simulink model "uz_pmsm_model_nonlinear"  (R2023a)
settings: Solver=FixedStepAuto  StartTime=0.0  StopTime=0.5  RelTol=1e-3
PreLoadFcn:
  | uz_pmsm_model_init_parameter
PostLoadFcn:
  | % Import the data from Excel for a lookup table
  | FluxMapData = readtable('C:\Users\Philipp\ultrazohm\ultrazohm_sw\ip_cores\uz_pmsm_model\FluxMapData_2023-05-26_13-07-57.csv');
  | % Row indices for lookup table
  | d_current_in_d_axis = FluxMapData(8:27,1:end);
  | % Column indices for lookup table
  | q_current_in_d_axis = FluxMapData(29:48,1:end);
  | % Output values for lookup table
  | d_Flux_d_axis = FluxMapData(50:69,1:end);
values from neighbouring files (symbols this model uses):
  d_current_d_Flux = FluxMapData{1,:}    [uz_pmsm_model_nonlinear_init_parameter.m]
  d_current_q_Flux = FluxMapData{66,:}    [uz_pmsm_model_nonlinear_init_parameter.m]
  Flux_d = FluxMapData{43:62,:}'*(1e-3)    [uz_pmsm_model_nonlinear_init_parameter.m]
  Flux_q = FluxMapData{108:end,:}'*(1e-3)    [uz_pmsm_model_nonlinear_init_parameter.m]
  friction_coefficient = 0.001    [uz_pmsm_model_nonlinear_init_parameter.m]
  inertia = 0.001    [uz_pmsm_model_nonlinear_init_parameter.m]
  k_i_d = R_1/(2*tau_sum)    (= 2812.5)    [uz_pmsm_model_nonlinear_init_parameter.m]
  k_p_d = L_d/(2*tau_sum)    (= 10.9375)    [uz_pmsm_model_nonlinear_init_parameter.m]
  k_p_q = L_q/(2*tau_sum)    (= 10.9375)    [uz_pmsm_model_nonlinear_init_parameter.m]
  L_d = 1.75e-3    (= 0.00175)    [uz_pmsm_model_nonlinear_init_parameter.m]
  L_q = 1.75e-3    (= 0.00175)    [uz_pmsm_model_nonlinear_init_parameter.m]
  polepair = 4    [uz_pmsm_model_nonlinear_init_parameter.m]
  psi_pm = 0.042    [uz_pmsm_model_nonlinear_init_parameter.m]
  q_current_d_Flux = FluxMapData{22:41,1}    [uz_pmsm_model_nonlinear_init_parameter.m]
  q_current_q_Flux = FluxMapData{87:106,1}    [uz_pmsm_model_nonlinear_init_parameter.m]
  R_1 = 0.45    [uz_pmsm_model_nonlinear_init_parameter.m]
  setpoint_step = 10.0    (= 10)    [compare_simulation_to_measurement.m]    (also in uz_pmsm_model_nonlinear_init_parameter.m)
  simulate_mechanical = true    [compare_simulation_to_measurement.m]    (also in uz_pmsm_model_nonlinear_init_parameter.m = false)
  simulate_open_loop = true    [compare_simulation_to_measurement.m]    (also in uz_pmsm_model_nonlinear_init_parameter.m)
  static_friction_torque = 0.01    [uz_pmsm_model_nonlinear_init_parameter.m]
  ts = 1/5e5    (= 2e-06)    [uz_pmsm_model_nonlinear_init_parameter.m]
undefined symbols (not defined in the file or in its folder): Ldd, Ldq, Lqd, Lqq
libraries: slpidlib x2
settings Model: DataTypeOverride=Off  Creator=ts  LastModifiedBy=Philipp
settings SolverCC: AlgebraicLoopSolver=TrustRegion  AutoInsertRateTranBlk=on
settings DataIOCC: LimitDataPoints=on  SaveOutput=off  SaveTime=off
settings OptimizationCC: BlockReduction=off  ConditionallyExecuteInputs=off  DefaultParameterBehavior=Inlined  LifeSpan=inf
settings DebuggingCC: AlgebraicLoopMsg=error  SingleTaskRateTransMsg=error  UnconnectedInputMsg=warning  UnconnectedOutputMsg=warning  UnconnectedLineMsg=warning  AllowSymbolicDim=off  StrictBusMsg=ErrorOnBusTreatedAsVector  SFUnexpectedBacktrackingDiag=warning  SFNoUnconditionalDefaultTransitionDiag=warning  SFExecutionAtInitializationDiag=none  ArithmeticOperatorsInVariantConditions=warning
settings HardwareCC: ProdBitPerPointer=32  ProdBitPerSizeT=32  ProdBitPerPtrDiffT=32  ProdLargestAtomicFloat=None  ProdIntDivRoundTo=Undefined  ProdEndianess=Unspecified  ProdWordSize=32  ProdHWDeviceType=ASIC/FPGA->ASIC/FPGA  ProdEqTarget=off
settings ModelReferenceCC: EnableRefExpFcnMdlSchedulingChecks=on
settings SFSimCC: SimUseLocalCustomCode=off  CustomCodeUndefinedFunction=UseInterfaceOnly
settings RTWCC: RTWUseLocalCustomCode=off  DLArmComputeVersion=19.05
settings CodeAppCC: StateflowObjectComments=on
settings GRTTargetCC: TargetLangStandard=C89/C90 (ANSI)
settings ConfigComp: CovScope=ReferencedModels  CovMetricSettings=dw  CovSaveCumulativeToWorkspaceVar=on  CovSaveSingleToWorkspaceVar=on  CovExternalEMLEnable=off  CovSFcnEnable=off

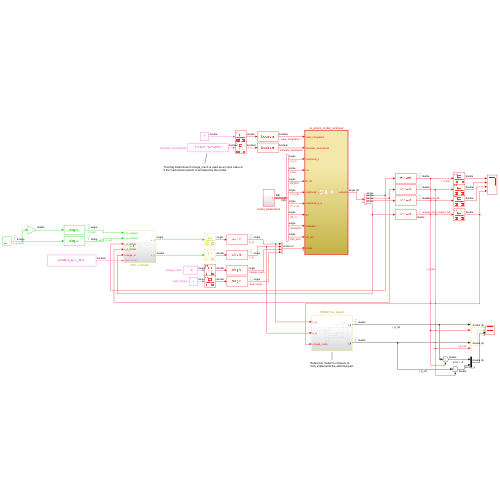
[thumbnail: Simulink's stored preview of the top-level diagram]
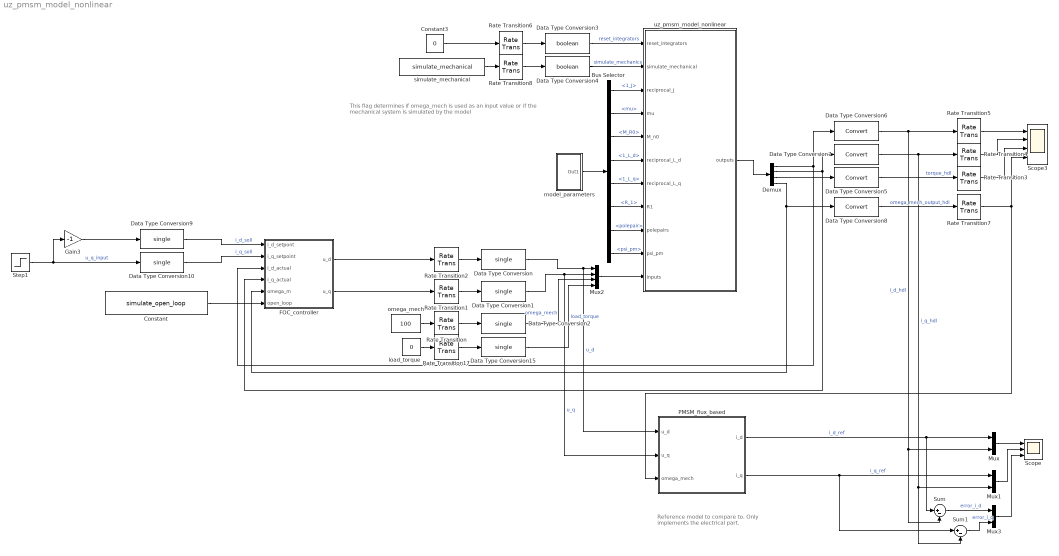
== system uz_pmsm_model_nonlinear ==
  note: Reference model to compare to.
      | Only implements the electrical part.
  note: This flag determines if omega_mech is used as an input value or
      | if the mechanical system is simulated by the model
  Bus Selector : BusSelector  OutputSignals=1_J,mu,M_R0,1_L_d,1_L_q,R_1,polepair,psi_pm
  Constant : Constant  Value=simulate_open_loop
  Constant3 : Constant  Value=0
  Data Type Conversion{,1..2,9..10,15} (6 alike) : DataTypeConversion  OutDataTypeStr=single  SaturateOnIntegerOverflow=off  RndMeth=Floor
  Data Type Conversion3 : DataTypeConversion  OutDataTypeStr=boolean  SaturateOnIntegerOverflow=off  RndMeth=Floor
  Data Type Conversion4 : DataTypeConversion  OutDataTypeStr=boolean  SaturateOnIntegerOverflow=off  RndMeth=Floor
  Data Type Conversion{5..8} (4 alike) : DataTypeConversion  SaturateOnIntegerOverflow=off  RndMeth=Floor
  Demux : Demux
  FOC_controller : Subsystem
  Gain3 : Gain  Gain=-1
  Mux : Mux  Inputs=2
  Mux1 : Mux  Inputs=2
  Mux2 : Mux
  Mux3 : Mux  Inputs=2
  PMSM_flux_based : Subsystem
  Rate Transition{,1..2,6,8,17} (6 alike) : RateTransition  OutPortSampleTime=ts
  Rate Transition{3..5,7} (4 alike) : RateTransition
  Scope : Scope  NumInputPorts=3
  Scope3 : Scope  NumInputPorts=4
  Step1 : Step  Time=0.2  After=setpoint_step
  Sum : Sum  Inputs=|+-
  Sum1 : Sum  Inputs=|+-
  load_torque : Constant  Value=0
  model_parameters : Subsystem
  omega_mech : Constant  Value=100
  simulate_mechanical : Constant  Value=simulate_mechanical
  uz_pmsm_model_nonlinear : Subsystem  TreatAsAtomicUnit=on
  wires:
  Rate Transition/1 -> Data Type Conversion2/1
  Rate Transition1/1 -> Data Type Conversion1/1
  Rate Transition2/1 -> Data Type Conversion/1
  Data Type Conversion6/1 -> Mux/2, Sum/2, Rate Transition5/1  "i_d_hdl"
  Data Type Conversion7/1 -> Rate Transition4/1, Mux1/2, Sum1/2  "i_q_hdl"
  Data Type Conversion5/1 -> Rate Transition3/1  "torque_hdl"
  Rate Transition4/1 -> Scope3/2
  Rate Transition5/1 -> Scope3/1
  Rate Transition3/1 -> Scope3/3
  Rate Transition6/1 -> Data Type Conversion3/1
  Constant3/1 -> Rate Transition6/1
  Rate Transition8/1 -> Data Type Conversion4/1
  simulate_mechanical/1 -> Rate Transition8/1
  Data Type Conversion3/1 -> uz_pmsm_model_nonlinear/1(reset_integrators)  "reset_integrators"
  Data Type Conversion4/1 -> uz_pmsm_model_nonlinear/2(simulate_mechanical)  "simulate_mechanics"
  load_torque/1 -> Rate Transition17/1
  Rate Transition17/1 -> Data Type Conversion15/1
  Mux/1 -> Scope/1
  Mux1/1 -> Scope/2
  PMSM_flux_based/2(i_q) -> Mux1/1, Sum1/1  "i_q_ref"
  PMSM_flux_based/1(i_d) -> Mux/1, Sum/1  "i_d_ref"
  Data Type Conversion8/1 -> Rate Transition7/1  "omega_mech_output_hdl"
  Rate Transition7/1 -> PMSM_flux_based/3(omega_mech), Scope3/4
  Bus Selector/1 -> uz_pmsm_model_nonlinear/3(reciprocal_J)  "<1_J>"
  Bus Selector/2 -> uz_pmsm_model_nonlinear/4(mu)  "<mu>"
  Bus Selector/3 -> uz_pmsm_model_nonlinear/5(M_n0)  "<M_R0>"
  Bus Selector/4 -> uz_pmsm_model_nonlinear/6(reciprocal_L_d)  "<1_L_d>"
  Bus Selector/5 -> uz_pmsm_model_nonlinear/7(reciprocal_L_q)  "<1_L_q>"
  Bus Selector/6 -> uz_pmsm_model_nonlinear/8(R1)  "<R_1>"
  Bus Selector/7 -> uz_pmsm_model_nonlinear/9(polepairs)  "<polepair>"
  Bus Selector/8 -> uz_pmsm_model_nonlinear/10(psi_pm)  "<psi_pm>"
  model_parameters/1(Out1) -> Bus Selector/1
  Sum/1 -> Mux3/1  "error_i_d"
  Sum1/1 -> Mux3/2  "error_i_q"
  Mux3/1 -> Scope/3
  Step1/1 -> Gain3/1, Data Type Conversion10/1  "u_q_input"
  Demux/3 -> Data Type Conversion5/1
  Gain3/1 -> Data Type Conversion9/1
  Demux/1 -> Data Type Conversion6/1, FOC_controller/3(i_d_actual)
  Demux/4 -> Data Type Conversion8/1, FOC_controller/5(omega_m)
  Demux/2 -> Data Type Conversion7/1, FOC_controller/4(i_q_actual)
  Data Type Conversion/1 -> PMSM_flux_based/1(u_d), Mux2/1  "u_d"
  Data Type Conversion1/1 -> PMSM_flux_based/2(u_q), Mux2/2  "u_q"
  Data Type Conversion15/1 -> Mux2/4  "load_torque"
  Data Type Conversion2/1 -> Mux2/3  "omega_mech"
  Mux2/1 -> uz_pmsm_model_nonlinear/11(inputs)
  uz_pmsm_model_nonlinear/1(outputs) -> Demux/1
  Data Type Conversion9/1 -> FOC_controller/1(i_d_setpont)  "i_d_soll"
  Data Type Conversion10/1 -> FOC_controller/2(i_q_setpoint)  "i_q_soll"
  FOC_controller/1(u_d) -> Rate Transition2/1
  FOC_controller/2(u_q) -> Rate Transition1/1
  omega_mech/1 -> Rate Transition/1
  Constant/1 -> FOC_controller/6(open_loop)

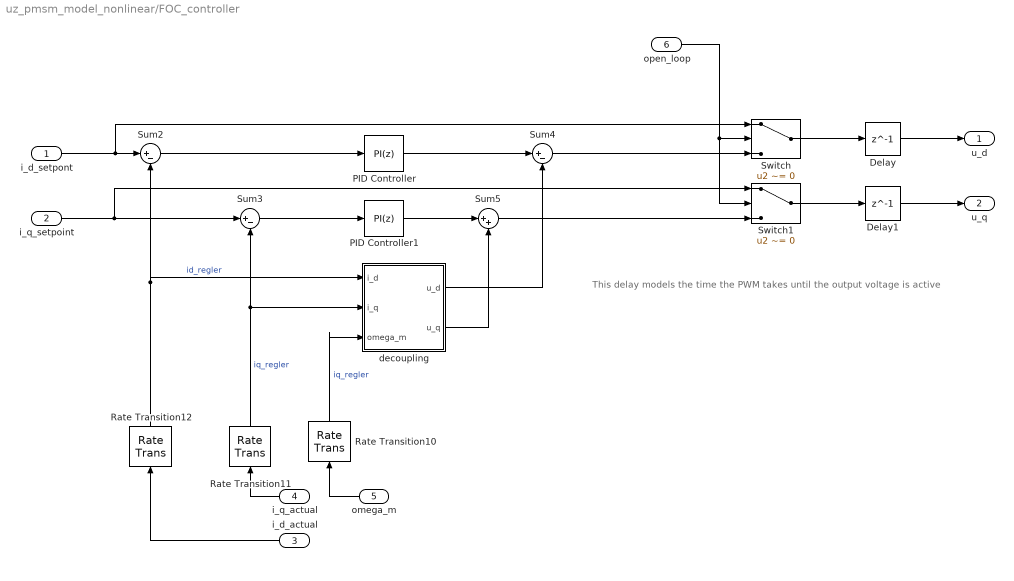
== system uz_pmsm_model_nonlinear/FOC_controller ==
  note: This delay models the time the PWM takes until the output voltage is active
  i_d_setpont : Inport
  i_q_setpoint : Inport  Port=2
  i_d_actual : Inport  Port=3
  i_q_actual : Inport  Port=4
  omega_m : Inport  Port=5
  open_loop : Inport  Port=6
  Delay : Delay  DelayLength=1
  Delay1 : Delay  DelayLength=1
  PID Controller : slpidlib/PID Controller  Controller=PI  Form=Parallel  TimeDomain=Discrete-time  UseExternalTs=off  SampleTime=-1  IntegratorMethod=Forward Euler  FilterMethod=Forward Euler  ControllerParametersSource=internal  P=k_p_d  I=k_i_d  UseKiTs=off  D=0  N=100  UseFilter=on  TunerSelectOption=Transfer Function Based (PID Tuner App)  InitialConditionSource=internal  InitialConditionForIntegrator=0  InitialConditionForFilter=0  DifferentiatorICPrevScaledInput=0  ExternalReset=none  TrackingMode=off  Kt=1  LimitOutput=off  SatLimitsSource=internal  UpperSaturationLimit=inf  LowerSaturationLimit=-inf  LinearizeAsGain=on  AntiWindupMode=none  Kb=1  LimitIntegrator=off  UpperIntegratorSaturationLimit=inf  LowerIntegratorSaturationLimit=-inf  POutMin=[]  POutMax=[]  IOutMin=[]  IOutMax=[]  DOutMin=[]  DOutMax=[]  NOutMin=[]  NOutMax=[]  SumOutMin=[]  SumOutMax=[]  SaturationOutMin=[]  SaturationOutMax=[]  PParamMin=[]  PParamMax=[]  IParamMin=[]  IParamMax=[]  DParamMin=[]  DParamMax=[]  NParamMin=[]  NParamMax=[]  KbParamMin=[]  KbParamMax=[]  KtParamMin=[]  KtParamMax=[]  KbOutMin=[]  KbOutMax=[]  KtOutMin=[]  KtOutMax=[]  IntegratorOutMin=[]  IntegratorOutMax=[]  FilterOutMin=[]  FilterOutMax=[]  SumI1OutMin=[]  SumI1OutMax=[]  SumI2OutMin=[]  SumI2OutMax=[]  SumI3OutMin=[]  SumI3OutMax=[]  SumI4OutMin=[]  SumI4OutMax=[]  SumDOutMin=[]  SumDOutMax=[]  DifferentiatorOutMin=[]  DifferentiatorOutMax=[]  FilterDiffOutCoefMin=[]  FilterDiffOutCoefMax=[]  ReciprocalOutMin=[]  ReciprocalOutMax=[]  SumDenOutMin=[]  SumDenOutMax=[]  SumNumOutMin=[]  SumNumOutMax=[]  DivideOutMin=[]  DivideOutMax=[]  UdiffTsProdOutMin=[]  UdiffTsProdOutMax=[]  NTsProdOutMin=[]  NTsProdOutMax=[]  UintegralTsProdOutMin=[]  UintegralTsProdOutMax=[]  UngainTsProdOutMin=[]  UngainTsProdOutMax=[]  ClampingZeroOutDataTypeStr=Inherit: Inherit via back propagation  ClampingZeroOutMin=[]  ClampingZeroOutMax=[]  FilterDenConstantOutDataTypeStr=Inherit: Inherit via back propagation  FilterDenConstantOutMin=[]  FilterDenConstantOutMax=[]  PCopyOutDataTypeStr=Inherit: Inherit via back propagation  PCopyOutMin=[]  PCopyOutMax=[]  NCopyOutDataTypeStr=Inherit: Inherit via back propagation  NCopyOutMin=[]  NCopyOutMax=[]  IntegratorContinuousStateAttributes=''  IntegratorStateMustResolveToSignalObject=off  IntegratorRTWStateStorageClass=Auto  FilterContinuousStateAttributes=''  FilterStateMustResolveToSignalObject=off  FilterRTWStateStorageClass=Auto  ParallelPVariant=InternalParameters  IdealPVariant=Disabled  IVariant=InternalParameters  DVariant=Disabled  IntegratorVariant=Discrete  SatVariant=Disabled  AWVariant=Passthrough  PCopyVariant=Disabled  TRVariant=Disabled  FdbkBlocksVariant=Forward  IdealPFdbkVariant=Disabled  SatFdbkVariant=Disabled  DerivativeFilterVariant=Disabled  NVariant=Disabled  NCopyVariant=Disabled_SignalSpec  FilterICVariant=Disabled  IntegratorICVariant=InternalICs  ExternalResetVariant=Disabled  TRSumVariant=Passthrough  SumFdbkVariant=Disabled  SumVariant=Sum_PI  TsampFilterVariant=InternalTs  TsampNgainVariant=Passthrough  TsampIntegralVariant=Disabled_SignalSpec  ExternalSaturationOutDataTypeStr=Inherit: Same as second input
  PID Controller1 : slpidlib/PID Controller  Controller=PI  Form=Parallel  TimeDomain=Discrete-time  UseExternalTs=off  SampleTime=-1  IntegratorMethod=Forward Euler  FilterMethod=Forward Euler  ControllerParametersSource=internal  P=k_p_q  I=k_i_d  UseKiTs=off  D=0  N=100  UseFilter=on  TunerSelectOption=Transfer Function Based (PID Tuner App)  InitialConditionSource=internal  InitialConditionForIntegrator=0  InitialConditionForFilter=0  DifferentiatorICPrevScaledInput=0  ExternalReset=none  TrackingMode=off  Kt=1  LimitOutput=off  SatLimitsSource=internal  UpperSaturationLimit=inf  LowerSaturationLimit=-inf  LinearizeAsGain=on  AntiWindupMode=none  Kb=1  LimitIntegrator=off  UpperIntegratorSaturationLimit=inf  LowerIntegratorSaturationLimit=-inf  POutMin=[]  POutMax=[]  IOutMin=[]  IOutMax=[]  DOutMin=[]  DOutMax=[]  NOutMin=[]  NOutMax=[]  SumOutMin=[]  SumOutMax=[]  SaturationOutMin=[]  SaturationOutMax=[]  PParamMin=[]  PParamMax=[]  IParamMin=[]  IParamMax=[]  DParamMin=[]  DParamMax=[]  NParamMin=[]  NParamMax=[]  KbParamMin=[]  KbParamMax=[]  KtParamMin=[]  KtParamMax=[]  KbOutMin=[]  KbOutMax=[]  KtOutMin=[]  KtOutMax=[]  IntegratorOutMin=[]  IntegratorOutMax=[]  FilterOutMin=[]  FilterOutMax=[]  SumI1OutMin=[]  SumI1OutMax=[]  SumI2OutMin=[]  SumI2OutMax=[]  SumI3OutMin=[]  SumI3OutMax=[]  SumI4OutMin=[]  SumI4OutMax=[]  SumDOutMin=[]  SumDOutMax=[]  DifferentiatorOutMin=[]  DifferentiatorOutMax=[]  FilterDiffOutCoefMin=[]  FilterDiffOutCoefMax=[]  ReciprocalOutMin=[]  ReciprocalOutMax=[]  SumDenOutMin=[]  SumDenOutMax=[]  SumNumOutMin=[]  SumNumOutMax=[]  DivideOutMin=[]  DivideOutMax=[]  UdiffTsProdOutMin=[]  UdiffTsProdOutMax=[]  NTsProdOutMin=[]  NTsProdOutMax=[]  UintegralTsProdOutMin=[]  UintegralTsProdOutMax=[]  UngainTsProdOutMin=[]  UngainTsProdOutMax=[]  ClampingZeroOutDataTypeStr=Inherit: Inherit via back propagation  ClampingZeroOutMin=[]  ClampingZeroOutMax=[]  FilterDenConstantOutDataTypeStr=Inherit: Inherit via back propagation  FilterDenConstantOutMin=[]  FilterDenConstantOutMax=[]  PCopyOutDataTypeStr=Inherit: Inherit via back propagation  PCopyOutMin=[]  PCopyOutMax=[]  NCopyOutDataTypeStr=Inherit: Inherit via back propagation  NCopyOutMin=[]  NCopyOutMax=[]  IntegratorContinuousStateAttributes=''  IntegratorStateMustResolveToSignalObject=off  IntegratorRTWStateStorageClass=Auto  FilterContinuousStateAttributes=''  FilterStateMustResolveToSignalObject=off  FilterRTWStateStorageClass=Auto  ParallelPVariant=InternalParameters  IdealPVariant=Disabled  IVariant=InternalParameters  DVariant=Disabled  IntegratorVariant=Discrete  SatVariant=Disabled  AWVariant=Passthrough  PCopyVariant=Disabled  TRVariant=Disabled  FdbkBlocksVariant=Forward  IdealPFdbkVariant=Disabled  SatFdbkVariant=Disabled  DerivativeFilterVariant=Disabled  NVariant=Disabled  NCopyVariant=Disabled_SignalSpec  FilterICVariant=Disabled  IntegratorICVariant=InternalICs  ExternalResetVariant=Disabled  TRSumVariant=Passthrough  SumFdbkVariant=Disabled  SumVariant=Sum_PI  TsampFilterVariant=InternalTs  TsampNgainVariant=Passthrough  TsampIntegralVariant=Disabled_SignalSpec  ExternalSaturationOutDataTypeStr=Inherit: Same as second input
  Rate Transition10 : RateTransition  OutPortSampleTime=ts_regler
  Rate Transition11 : RateTransition  OutPortSampleTime=ts_regler
  Rate Transition12 : RateTransition  OutPortSampleTime=ts_regler
  Sum2 : Sum  Inputs=|+-
  Sum3 : Sum  Inputs=|+-
  Sum4 : Sum  Inputs=|+-
  Sum5 : Sum  Inputs=|++
  Switch : Switch  Criteria=u2 ~= 0  SaturateOnIntegerOverflow=off  InputSameDT=off
  Switch1 : Switch  Criteria=u2 ~= 0  SaturateOnIntegerOverflow=off  InputSameDT=off
  decoupling : Subsystem
  u_d : Outport
  u_q : Outport  Port=2
  wires:
  PID Controller/1 -> Sum4/1
  PID Controller1/1 -> Sum5/1
  Sum4/1 -> Switch/3
  i_d_actual/1 -> Rate Transition12/1
  i_d_setpont/1 -> Switch/1, Sum2/1
  Sum2/1 -> PID Controller/1
  Sum5/1 -> Switch1/3
  omega_m/1 -> Rate Transition10/1
  Sum3/1 -> PID Controller1/1
  i_q_actual/1 -> Rate Transition11/1
  Rate Transition12/1 -> decoupling/1(i_d), Sum2/2  "id_regler"
  Rate Transition11/1 -> decoupling/2(i_q), Sum3/2  "iq_regler"
  i_q_setpoint/1 -> Switch1/1, Sum3/1
  open_loop/1 -> Switch1/2, Switch/2
  Rate Transition10/1 -> decoupling/3(omega_m)  "iq_regler"
  decoupling/1(u_d) -> Sum4/2
  decoupling/2(u_q) -> Sum5/2
  Switch/1 -> Delay/1
  Switch1/1 -> Delay1/1
  Delay/1 -> u_d/1
  Delay1/1 -> u_q/1

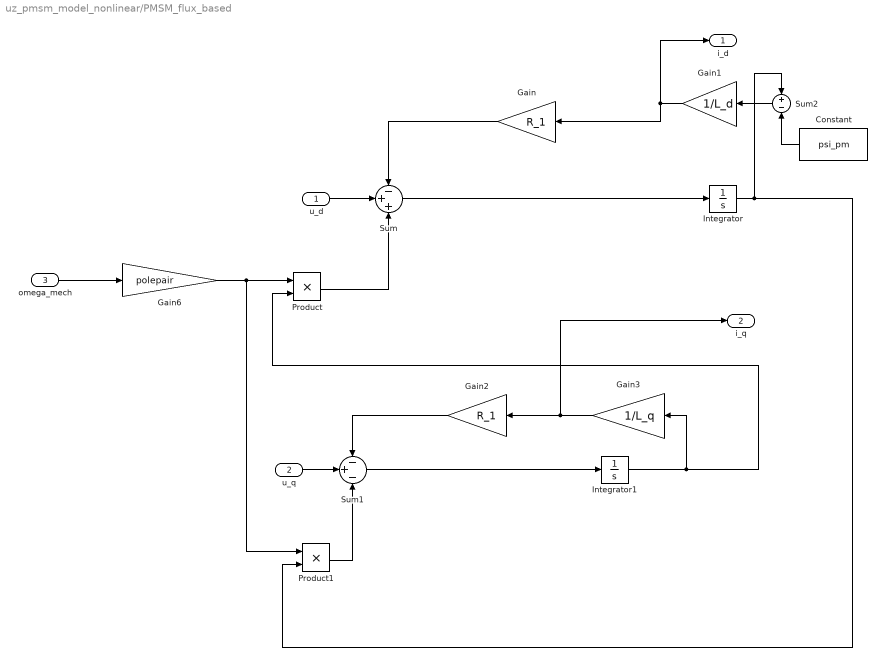
== system uz_pmsm_model_nonlinear/PMSM_flux_based ==
  u_d : Inport
  u_q : Inport  Port=2
  omega_mech : Inport  Port=3
  Constant : Constant  Value=psi_pm
  Gain : Gain  Gain=R_1
  Gain1 : Gain  Gain=1/L_d
  Gain2 : Gain  Gain=R_1
  Gain3 : Gain  Gain=1/L_q
  Gain6 : Gain  Gain=polepair
  Integrator : Integrator
  Integrator1 : Integrator
  Product : Product
  Product1 : Product
  Sum : Sum  Inputs=-++
  Sum1 : Sum  Inputs=-+-
  Sum2 : Sum  Inputs=+-
  i_d : Outport
  i_q : Outport  Port=2
  wires:
  u_d/1 -> Sum/2
  u_q/1 -> Sum1/2
  Sum/1 -> Integrator/1
  Gain/1 -> Sum/1
  Integrator/1 -> Product1/2, Sum2/1
  Constant/1 -> Sum2/2
  Sum2/1 -> Gain1/1
  Gain1/1 -> Gain/1, i_d/1
  Gain6/1 -> Product1/1, Product/1
  Product/1 -> Sum/3
  Integrator1/1 -> Gain3/1, Product/2
  Product1/1 -> Sum1/3
  Sum1/1 -> Integrator1/1
  Gain2/1 -> Sum1/1
  Gain3/1 -> i_q/1, Gain2/1
  omega_mech/1 -> Gain6/1

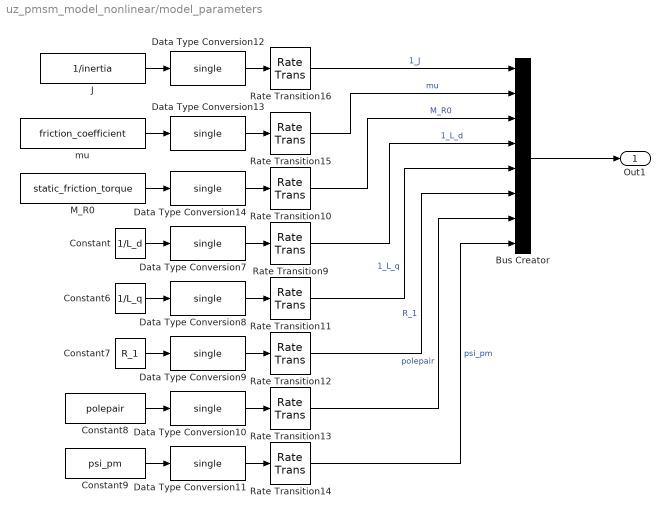
== system uz_pmsm_model_nonlinear/model_parameters ==
  Bus Creator : BusCreator  Inputs=8
  Constant : Constant  Value=1/L_d
  Constant6 : Constant  Value=1/L_q
  Constant7 : Constant  Value=R_1
  Constant8 : Constant  Value=polepair
  Constant9 : Constant  Value=psi_pm
  Data Type Conversion{7..14} (8 alike) : DataTypeConversion  OutDataTypeStr=single  SaturateOnIntegerOverflow=off  RndMeth=Floor
  J : Constant  Value=1/inertia
  M_R0 : Constant  Value=static_friction_torque
  Rate Transition{9..16} (8 alike) : RateTransition  OutPortSampleTime=ts
  mu : Constant  Value=friction_coefficient
  Out1 : Outport
  wires:
  Data Type Conversion12/1 -> Rate Transition16/1
  Data Type Conversion7/1 -> Rate Transition9/1
  Rate Transition10/1 -> Bus Creator/3  "M_R0"
  Rate Transition14/1 -> Bus Creator/8  "psi_pm"
  Data Type Conversion14/1 -> Rate Transition10/1
  Rate Transition12/1 -> Bus Creator/6  "R_1"
  Rate Transition16/1 -> Bus Creator/1  "1_J"
  Rate Transition13/1 -> Bus Creator/7  "polepair"
  Bus Creator/1 -> Out1/1
  Data Type Conversion11/1 -> Rate Transition14/1
  Constant8/1 -> Data Type Conversion10/1
  Data Type Conversion9/1 -> Rate Transition12/1
  Rate Transition15/1 -> Bus Creator/2  "mu"
  Constant6/1 -> Data Type Conversion8/1
  Rate Transition9/1 -> Bus Creator/4  "1_L_d"
  J/1 -> Data Type Conversion12/1
  Data Type Conversion8/1 -> Rate Transition11/1
  Data Type Conversion10/1 -> Rate Transition13/1
  mu/1 -> Data Type Conversion13/1
  M_R0/1 -> Data Type Conversion14/1
  Rate Transition11/1 -> Bus Creator/5  "1_L_q"
  Data Type Conversion13/1 -> Rate Transition15/1
  Constant7/1 -> Data Type Conversion9/1
  Constant9/1 -> Data Type Conversion11/1
  Constant/1 -> Data Type Conversion7/1

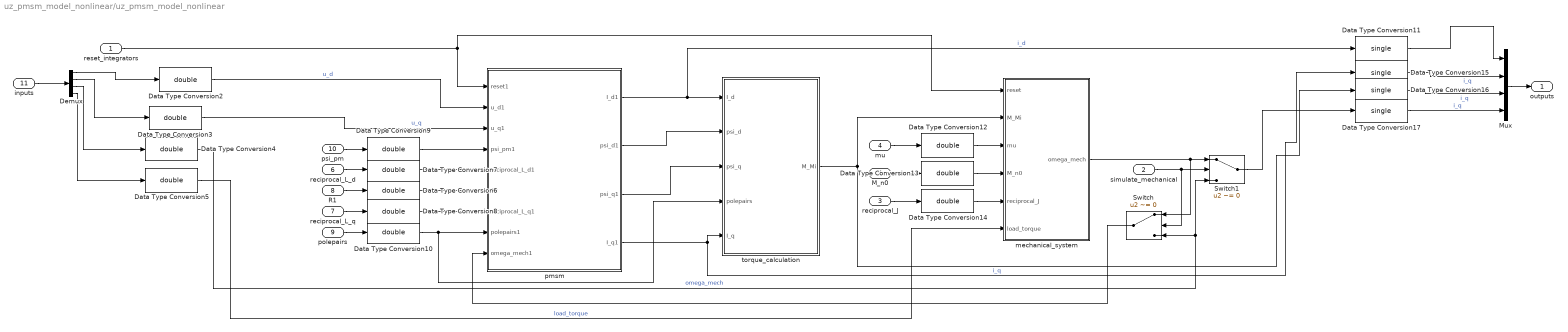
== system uz_pmsm_model_nonlinear/uz_pmsm_model_nonlinear ==
  reset_integrators : Inport
  simulate_mechanical : Inport  Port=2
  reciprocal_J : Inport  Port=3
  mu : Inport  Port=4
  M_n0 : Inport  Port=5
  reciprocal_L_d : Inport  Port=6
  reciprocal_L_q : Inport  Port=7
  R1 : Inport  Port=8
  polepairs : Inport  Port=9
  psi_pm : Inport  Port=10
  inputs : Inport  Port=11
  Data Type Conversion{2..10,12..14} (12 alike) : DataTypeConversion  OutDataTypeStr=double  RndMeth=Nearest  SaturateOnIntegerOverflow=off
  Data Type Conversion{11,15..17} (4 alike) : DataTypeConversion  OutDataTypeStr=single  RndMeth=Nearest  SaturateOnIntegerOverflow=off
  Demux : Demux
  Mux : Mux
  Switch : Switch  Criteria=u2 ~= 0  SaturateOnIntegerOverflow=off  InputSameDT=off
  Switch1 : Switch  Criteria=u2 ~= 0  SaturateOnIntegerOverflow=off  InputSameDT=off
  mechanical_system : Subsystem
  pmsm : Subsystem
  torque_calculation : Subsystem
  outputs : Outport
  wires:
  reset_integrators/1 -> pmsm/1(reset1), mechanical_system/1(reset)
  Data Type Conversion4/1 -> Switch1/3, Switch/3  "omega_mech"
  Switch/1 -> pmsm/9(omega_mech1)
  reciprocal_J/1 -> Data Type Conversion14/1
  pmsm/2(psi_d1) -> torque_calculation/2(psi_d)
  Data Type Conversion5/1 -> mechanical_system/6(load_torque)  "load_torque"
  Data Type Conversion7/1 -> pmsm/5(reciprocal_L_d1)
  Switch1/1 -> Data Type Conversion17/1
  Data Type Conversion9/1 -> pmsm/4(psi_pm1)
  R1/1 -> Data Type Conversion6/1
  Data Type Conversion6/1 -> pmsm/6(R2)
  pmsm/3(psi_q1) -> torque_calculation/3(psi_q)
  Data Type Conversion10/1 -> pmsm/8(polepairs1), torque_calculation/4(polepairs)
  Data Type Conversion2/1 -> pmsm/2(u_d1)  "u_d"
  Data Type Conversion12/1 -> mechanical_system/3(mu)
  simulate_mechanical/1 -> Switch1/2, Switch/2
  M_n0/1 -> Data Type Conversion13/1
  Data Type Conversion14/1 -> mechanical_system/5(reciprocal_J)
  torque_calculation/1(M_Mi) -> mechanical_system/2(M_Mi), Data Type Conversion16/1
  mu/1 -> Data Type Conversion12/1
  psi_pm/1 -> Data Type Conversion9/1
  Data Type Conversion13/1 -> mechanical_system/4(M_n0)
  reciprocal_L_d/1 -> Data Type Conversion7/1
  Data Type Conversion8/1 -> pmsm/7(reciprocal_L_q1)
  reciprocal_L_q/1 -> Data Type Conversion8/1
  polepairs/1 -> Data Type Conversion10/1
  Data Type Conversion3/1 -> pmsm/3(u_q1)  "u_q"
  mechanical_system/1(omega_mech) -> Switch/1, Switch1/1
  pmsm/4(I_q1) -> torque_calculation/5(I_q), Data Type Conversion15/1  "i_q"
  pmsm/1(I_d1) -> Data Type Conversion11/1, torque_calculation/1(I_d)  "i_d"
  Data Type Conversion17/1 -> Mux/4  "i_q"
  Data Type Conversion16/1 -> Mux/3  "i_q"
  Data Type Conversion15/1 -> Mux/2  "i_q"
  Data Type Conversion11/1 -> Mux/1
  Demux/1 -> Data Type Conversion2/1
  Demux/2 -> Data Type Conversion3/1
  Demux/3 -> Data Type Conversion4/1
  Demux/4 -> Data Type Conversion5/1
  inputs/1 -> Demux/1
  Mux/1 -> outputs/1

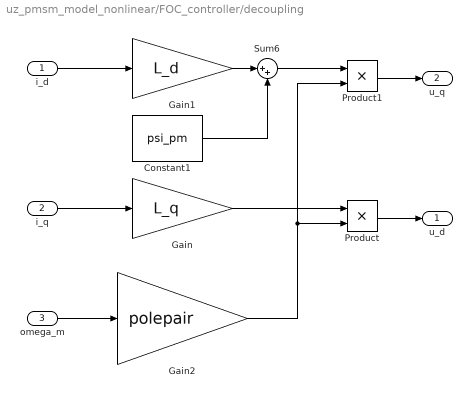
== system uz_pmsm_model_nonlinear/FOC_controller/decoupling ==
  i_d : Inport
  i_q : Inport  Port=2
  omega_m : Inport  Port=3
  Constant1 : Constant  Value=psi_pm  SampleTime=-1
  Gain : Gain  Gain=L_q
  Gain1 : Gain  Gain=L_d
  Gain2 : Gain  Gain=polepair
  Product : Product
  Product1 : Product
  Sum6 : Sum  Inputs=|++
  u_d : Outport
  u_q : Outport  Port=2
  wires:
  Gain/1 -> Product/1
  Gain2/1 -> Product1/2, Product/2
  Product1/1 -> u_q/1
  i_d/1 -> Gain1/1
  Product/1 -> u_d/1
  Gain1/1 -> Sum6/1
  i_q/1 -> Gain/1
  Constant1/1 -> Sum6/2
  Sum6/1 -> Product1/1
  omega_m/1 -> Gain2/1

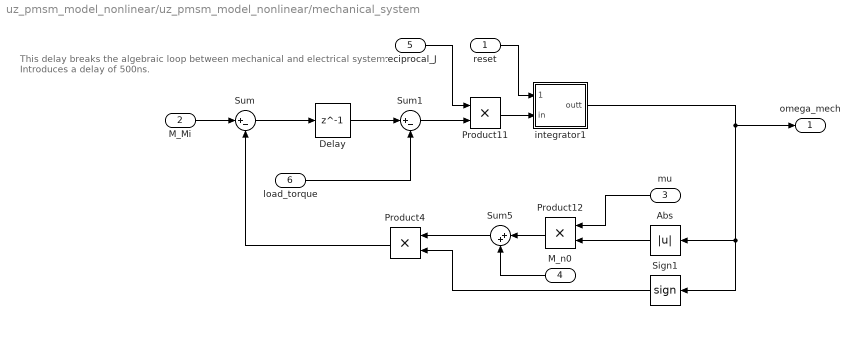
== system uz_pmsm_model_nonlinear/uz_pmsm_model_nonlinear/mechanical_system ==
  note: This delay breaks the algebraic loop between mechanical and electrical system.
      | Introduces a delay of 500ns.
  reset : Inport
  M_Mi : Inport  Port=2
  mu : Inport  Port=3
  M_n0 : Inport  Port=4
  reciprocal_J : Inport  Port=5
  load_torque : Inport  Port=6
  Abs : Abs  SaturateOnIntegerOverflow=off
  Delay : Delay  DelayLength=1
  Product11 : Product
  Product12 : Product
  Product4 : Product
  Sign1 : Signum
  Sum : Sum  Inputs=|+-
  Sum1 : Sum  Inputs=|+-
  Sum5 : Sum  Inputs=|++
  integrator1 : Subsystem
  omega_mech : Outport
  wires:
  Product11/1 -> integrator1/2(in)
  Sum5/1 -> Product4/1
  Sign1/1 -> Product4/2
  integrator1/1(outt) -> Sign1/1, Abs/1, omega_mech/1
  Abs/1 -> Product12/2
  reset/1 -> integrator1/1(reset)
  Product12/1 -> Sum5/1
  mu/1 -> Product12/1
  M_n0/1 -> Sum5/2
  reciprocal_J/1 -> Product11/1
  M_Mi/1 -> Sum/1
  Sum1/1 -> Product11/2
  load_torque/1 -> Sum1/2
  Sum/1 -> Delay/1
  Product4/1 -> Sum/2
  Delay/1 -> Sum1/1

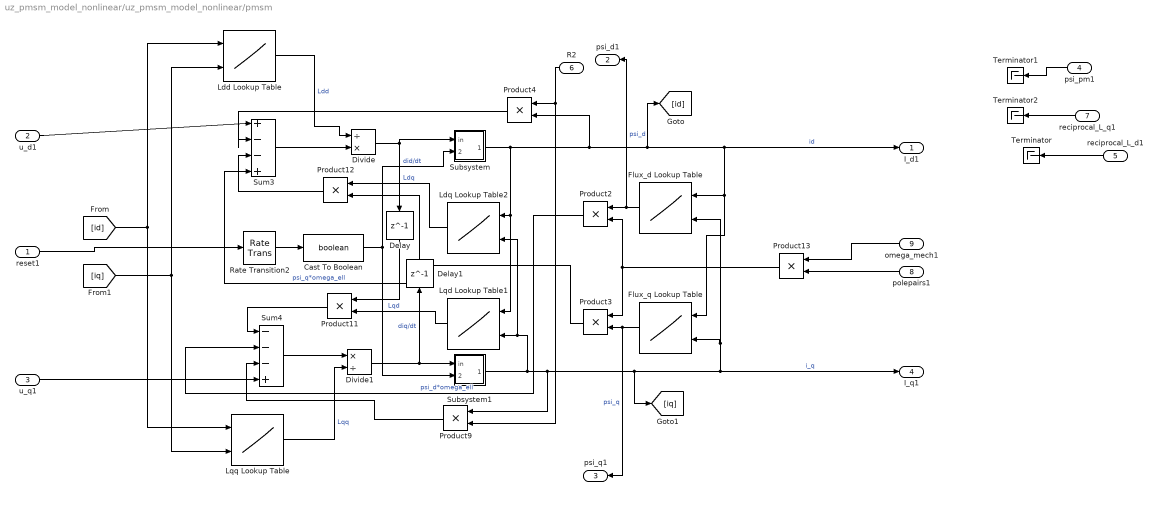
== system uz_pmsm_model_nonlinear/uz_pmsm_model_nonlinear/pmsm ==
  reset1 : Inport
  u_d1 : Inport  Port=2
  u_q1 : Inport  Port=3
  psi_pm1 : Inport  Port=4
  reciprocal_L_d1 : Inport  Port=5
  R2 : Inport  Port=6
  reciprocal_L_q1 : Inport  Port=7
  polepairs1 : Inport  Port=8
  omega_mech1 : Inport  Port=9
  Cast To Boolean : DataTypeConversion  OutDataTypeStr=boolean  SaturateOnIntegerOverflow=off  RndMeth=Floor
  Delay : Delay  DelayLength=1
  Delay1 : Delay  DelayLength=1
  Divide : Product  Inputs=/*
  Divide1 : Product  Inputs=*/
  Flux_d Lookup Table : Lookup_n-D  BreakpointsForDimension1=d_current_d_Flux  BreakpointsForDimension2=q_current_d_Flux  BreakpointsForDimension3=[5, 7]  Table=Flux_d  InternalRulePriority=Speed  RndMeth=Simplest
      settings: InputPortMap=u0,u1
  Flux_q Lookup Table : Lookup_n-D  BreakpointsForDimension1=d_current_q_Flux  BreakpointsForDimension2=q_current_q_Flux  BreakpointsForDimension3=[5, 7]  Table=Flux_q  InternalRulePriority=Speed  RndMeth=Simplest
      settings: InputPortMap=u0,u1
  Ldd Lookup Table : Lookup_n-D  BreakpointsForDimension1=d_current_q_Flux  BreakpointsForDimension2=q_current_q_Flux  BreakpointsForDimension3=[5, 7]  Table=Ldd  InternalRulePriority=Speed  RndMeth=Simplest
      settings: InputPortMap=u0,u1
  Ldq Lookup Table2 : Lookup_n-D  BreakpointsForDimension1=d_current_q_Flux  BreakpointsForDimension2=q_current_q_Flux  BreakpointsForDimension3=[5, 7]  Table=Ldq  InternalRulePriority=Speed  RndMeth=Simplest
      settings: InputPortMap=u0,u1
  Lqd Lookup Table1 : Lookup_n-D  BreakpointsForDimension1=d_current_q_Flux  BreakpointsForDimension2=q_current_q_Flux  BreakpointsForDimension3=[5, 7]  Table=Lqd  InternalRulePriority=Speed  RndMeth=Simplest
      settings: InputPortMap=u0,u1
  Lqq Lookup Table : Lookup_n-D  BreakpointsForDimension1=d_current_q_Flux  BreakpointsForDimension2=q_current_q_Flux  BreakpointsForDimension3=[5, 7]  Table=Lqq  InternalRulePriority=Speed  RndMeth=Simplest
      settings: InputPortMap=u0,u1
  Product{2..4,9,11..13} (7 alike) : Product
  Rate Transition2 : RateTransition  OutPortSampleTime=ts
  Subsystem : Subsystem
  Subsystem1 : Subsystem
  Sum3 : Sum  Inputs=|+--+
  Sum4 : Sum  Inputs=|---+
  Terminator : Terminator
  Terminator1 : Terminator
  Terminator2 : Terminator
  I_d1 : Outport
  psi_d1 : Outport  Port=2
  psi_q1 : Outport  Port=3
  I_q1 : Outport  Port=4
  wires:
  Ldq Lookup Table2/1 -> Product12/1  "Ldq"
  Sum4/1 -> Divide1/1
  u_q1/1 -> Sum4/4
  omega_mech1/1 -> Product13/1
  reciprocal_L_d1/1 -> Terminator/1
  Divide1/1 -> Subsystem1/1(in), Delay1/1  "diq/dt"
  polepairs1/1 -> Product13/2
  Lqd Lookup Table1/1 -> Product11/2  "Lqd"
  Product13/1 -> Product2/2, Product3/1
  Flux_d Lookup Table/1 -> psi_d1/1, Product2/1  "psi_d"
  Product12/1 -> Sum3/3
  Divide/1 -> Delay/1, Subsystem/1(in)  "did/dt"
  Sum3/1 -> Divide/2
  Product9/1 -> Sum4/3
  Cast To Boolean/1 -> Subsystem/2(reset), Subsystem1/2(reset)
  u_d1/1 -> Sum3/1
  reset1/1 -> Rate Transition2/1
  Product11/1 -> Sum4/1
  reciprocal_L_q1/1 -> Terminator2/1
  Rate Transition2/1 -> Cast To Boolean/1
  R2/1 -> Product9/2, Product4/1
  Subsystem/1(outt) -> Ldq Lookup Table2/1, Lqd Lookup Table1/1, Product4/2, I_d1/1, Flux_d Lookup Table/1, Flux_q Lookup Table/1, [id]  "id"
  [id] -> Lqq Lookup Table/1, Ldd Lookup Table/1
  Ldd Lookup Table/1 -> Divide/1  "Ldd"
  psi_pm1/1 -> Terminator1/1
  Subsystem1/1(outt) -> Ldq Lookup Table2/2, Lqd Lookup Table1/2, Product9/1, [iq], I_q1/1, Flux_q Lookup Table/2, Flux_d Lookup Table/2  "i_q"
  [iq] -> Ldd Lookup Table/2, Lqq Lookup Table/2
  Flux_q Lookup Table/1 -> psi_q1/1, Product3/2  "psi_q"
  Product3/1 -> Sum3/4  "psi_q*omega_ell"
  Lqq Lookup Table/1 -> Divide1/2  "Lqq"
  Product4/1 -> Sum3/2
  Product2/1 -> Sum4/2  "psi_d*omega_ell"
  Delay/1 -> Product11/1
  Delay1/1 -> Product12/2

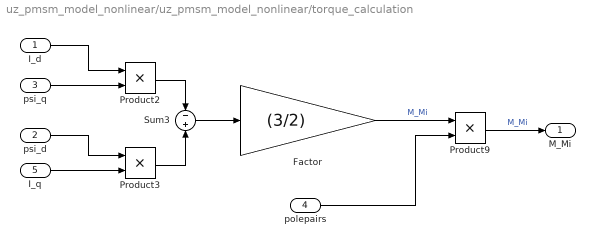
== system uz_pmsm_model_nonlinear/uz_pmsm_model_nonlinear/torque_calculation ==
  I_d : Inport
  psi_d : Inport  Port=2
  psi_q : Inport  Port=3
  polepairs : Inport  Port=4
  I_q : Inport  Port=5
  Factor : Gain  Gain=(3/2)
  Product2 : Product
  Product3 : Product
  Product9 : Product
  Sum3 : Sum  Inputs=-|+
  M_Mi : Outport
  wires:
  Sum3/1 -> Factor/1
  Product3/1 -> Sum3/2
  Product2/1 -> Sum3/1
  psi_q/1 -> Product2/2
  psi_d/1 -> Product3/1
  I_d/1 -> Product2/1
  I_q/1 -> Product3/2
  Product9/1 -> M_Mi/1  "M_Mi"
  polepairs/1 -> Product9/2
  Factor/1 -> Product9/1  "M_Mi"

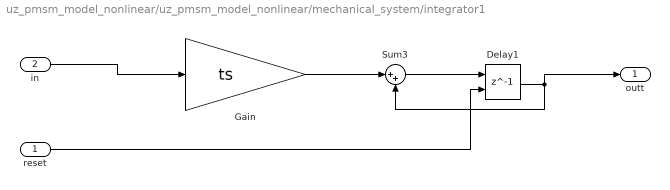
== system uz_pmsm_model_nonlinear/uz_pmsm_model_nonlinear/mechanical_system/integrator1 ==
  reset : Inport
  in : Inport  Port=2
  Delay1 : Delay  DelayLength=1  ExternalReset=Level
      settings: InputPortMap=u0,r5
  Gain : Gain  Gain=ts  OutDataTypeStr=double
  Sum3 : Sum  Inputs=|++  OutDataTypeStr=double
  outt : Outport
  wires:
  in/1 -> Gain/1
  Gain/1 -> Sum3/1
  reset/1 -> Delay1/2
  Sum3/1 -> Delay1/1
  Delay1/1 -> Sum3/2, outt/1

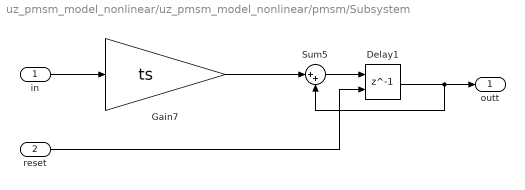
== system uz_pmsm_model_nonlinear/uz_pmsm_model_nonlinear/pmsm/Subsystem ==
  in : Inport
  reset : Inport  Port=2
  Delay1 : Delay  DelayLength=1  ExternalReset=Level
      settings: InputPortMap=u0,r5
  Gain7 : Gain  Gain=ts  OutDataTypeStr=double
  Sum5 : Sum  Inputs=|++  OutDataTypeStr=double
  outt : Outport
  wires:
  in/1 -> Gain7/1
  reset/1 -> Delay1/2
  Delay1/1 -> outt/1, Sum5/2
  Gain7/1 -> Sum5/1
  Sum5/1 -> Delay1/1

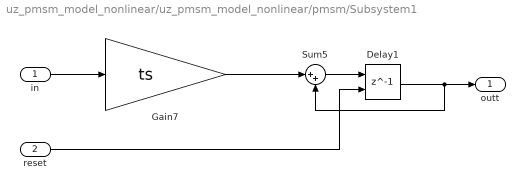
== system uz_pmsm_model_nonlinear/uz_pmsm_model_nonlinear/pmsm/Subsystem1 ==
  in : Inport
  reset : Inport  Port=2
  Delay1 : Delay  DelayLength=1  ExternalReset=Level
      settings: InputPortMap=u0,r5
  Gain7 : Gain  Gain=ts  OutDataTypeStr=double
  Sum5 : Sum  Inputs=|++  OutDataTypeStr=double
  outt : Outport
  wires:
  in/1 -> Gain7/1
  reset/1 -> Delay1/2
  Delay1/1 -> outt/1, Sum5/2
  Gain7/1 -> Sum5/1
  Sum5/1 -> Delay1/1
